simulink model "SimplePendulumWithFeedback"  (R2014a)
settings: Solver=ode45  StartTime=0.0  StopTime=T  RelTol=1e-3
undefined symbols (not defined in the file): b, den, g, Jr, m, num, r, theta0, thetaBar
settings Model: Creator=mauricio  LastModifiedBy=mauricio
settings DataIOCC: SignalLoggingSaveFormat=ModelDataLogs
settings OptimizationCC: ExpressionDepthLimit=2147483647
settings DebuggingCC: UnderspecifiedInitializationDetection=Classic  SolverPrmCheckMsg=none  FcnCallInpInsideContextMsg=UseLocalSettings  StateNameClashWarn=warning
settings GRTTargetCC: CombineOutputUpdateFcns=off  GRTInterface=on

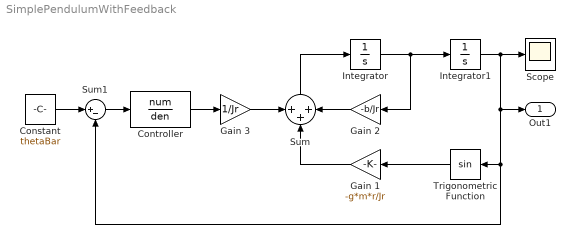
== system SimplePendulumWithFeedback ==
  Constant : Constant  Value=thetaBar
  Controller : TransferFcn  Numerator=num  Denominator=den
  Gain 1 : Gain  Gain=-g*m*r/Jr
  Gain 2 : Gain  Gain=-b/Jr
  Gain 3 : Gain  Gain=1/Jr
  Integrator : Integrator
  Integrator1 : Integrator  InitialCondition=theta0
  Scope : Scope
      settings: YMin=-3.141592653589793  YMax=3.141592653589793
  Sum : Sum  Inputs=+++
  Sum1 : Sum  Inputs=|+-
  Trigonometric Function : Trigonometry
  Out1 : Outport
  wires:
  Integrator/1 -> Integrator1/1, Gain 2/1
  Integrator1/1 -> Scope/1, Trigonometric Function/1, Sum1/2, Out1/1
  Trigonometric Function/1 -> Gain 1/1
  Sum/1 -> Integrator/1
  Gain 2/1 -> Sum/3
  Gain 1/1 -> Sum/2
  Sum1/1 -> Controller/1
  Controller/1 -> Gain 3/1
  Constant/1 -> Sum1/1
  Gain 3/1 -> Sum/1
